simulink model "Center_tapped_fw_rectifier"  (R2024b)
settings: Solver=VariableStepAuto  StartTime=0.0  StopTime=0.05  RelTol=1e-3
libraries: spsDiodeLib x2, spsGroundLib x2, spsVoltageMeasurementLib x2, spsParallelRLCBranchLib x1, spsACVoltageSourceLib x1, spsLinearTransformerLib x1, spsCurrentMeasurementLib x1, sps_lib x1
settings Model: Creator=PRASHANTH  LastModifiedBy=PRASHANTH

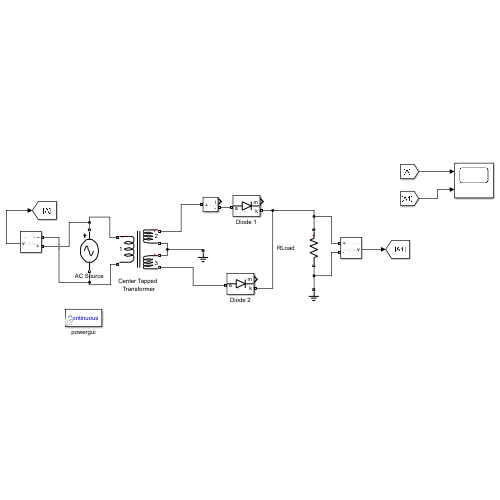
[thumbnail: Simulink's stored preview of the top-level diagram]
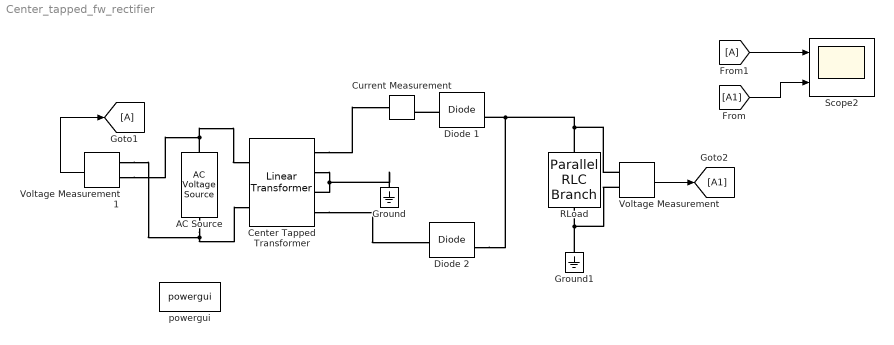
== system Center_tapped_fw_rectifier ==
  "   RLoad" : spsParallelRLCBranchLib/Parallel RLC Branch  LConnTagsString=a  RConnTagsString=__new0  BranchType=R  Resistance=10  Inductance=1e-3  SetiL0=off  InitialCurrent=0  Capacitance=1e-6  Setx0=off  InitialVoltage=0  Measurements=None
  AC Source : spsACVoltageSourceLib/AC Voltage Source  Amplitude=312  Phase=0  Frequency=50  SampleTime=0  Measurements=None  BusType=swing  Pref=10e3  Qref=0  Qmin=-inf  Qmax=+inf
  Center Tapped Transformer : spsLinearTransformerLib/Linear Transformer  UNITS=pu  NominalPower=[ 250e6 50 ]  winding1="[ 312  0.002  0.08 ]"  winding2="[ 312  0.002  0.08 ]"  ThreeWindings=on  winding3="[ 312  0.002  0.08 ]"  RmLm=[ 500 500 ]  Measurements=None  DataType=off
  Current Measurement : spsCurrentMeasurementLib/Current Measurement  PhasorSimulation=off  OutputType=Complex  PSBequivalent=0
  Diode 1 : spsDiodeLib/Diode  Ron=0.001  Lon=0  Vf=0.8  IC=0  UseSnubber=0  Rs=500  Cs=0  Measurements=on
  Diode 2 : spsDiodeLib/Diode  Ron=0.001  Lon=0  Vf=0.8  IC=0  UseSnubber=0  Rs=500  Cs=0  Measurements=on
  From1 : From
  Goto1 : Goto
  Ground : spsGroundLib/Ground  LConnTagsString=a
  Ground1 : spsGroundLib/Ground  LConnTagsString=a
  Scope2 : Scope  NumInputPorts=2
  Voltage Measurement : spsVoltageMeasurementLib/Voltage Measurement  PhasorSimulation=off  OutputType=Complex  PSBequivalent=0
  Voltage Measurement1 : spsVoltageMeasurementLib/Voltage Measurement  PhasorSimulation=off  OutputType=Complex  PSBequivalent=0
  powergui : sps_lib/powergui  Priority=1  SimulationMode=Continuous  SampleTime=50e-6  frequency=60  Iterations=50  frequencyindice=50  Pbase=100e6  ErrMax=1e-4  UnitsV=kV  UnitsW=MW  buscounter=0  FunctionMessages=off  echomessages=off  EnableUseOfTLC=off  CurrentSourceSwitches=off  DisableSnubberDevices=off  DisableRonSwitches=off  DisableVfSwitches=off  DisplayEquations=off  AutomaticDiscreteSolvers=off  SolverType=Tustin/Backward Euler (TBE)  Interpol=off  ExternalGateDelay=off  methode=off  Ts=100  x0status=blocks  SPID=on  SwTol=0  HookPort=off  NonlinearTolerance=1e-4  nMaxIteration=100  ContinueOnMaxIteration=off  RestoreLinks=warning  ResistiveCurrentMeasurement=off  Frange=[0:2:500]  Ylog=off  Xlog=on  ShowGrid=off  save=off  variable=ZData  structure=0  ZoomFFT=off  StartTime=0.0  cycles=1  DisplayStyle=1  fundamental=60  FreqAxis=off  MaxFrequency=1000  frequencyindicesteady=1  RmsSteady=1  display=off
  wires:
  Voltage Measurement/1 -> [A1]
  [A1] -> Scope2/2
  From1/1 -> Scope2/1
  Voltage Measurement1/1 -> Goto1/1
  connections:
  AC Source/RConn1 -- Center Tapped Transformer/LConn1 -- Voltage Measurement1/LConn1
  AC Source/LConn1 -- Voltage Measurement1/LConn2 -- Center Tapped Transformer/LConn2
  Diode 1/LConn1 -- Current Measurement/RConn1
  Voltage Measurement/LConn1 -- "   RLoad"/LConn1 -- Diode 2/RConn1 -- Diode 1/RConn1
  Voltage Measurement/LConn2 -- "   RLoad"/RConn1 -- Ground1/LConn1
  Center Tapped Transformer/RConn1 -- Current Measurement/LConn1
  Center Tapped Transformer/RConn2 -- Ground/LConn1 -- Center Tapped Transformer/RConn3
  Center Tapped Transformer/RConn4 -- Diode 2/LConn1
